simulink model "SIMbuckconverterPVmodel"  (R2020b)
settings: Solver=VariableStepAuto  StartTime=0.0  StopTime=3  RelTol=1e-3
libraries: powerlib x10, pid_lib x1, simulink x1
settings Model: SILPILModeSetting=veronly  ExtModeTrigDuration=2  Creator=colpari  LastModifiedBy=colpari
settings OptimizationCC: EnhancedBackFolding=on  PassReuseOutputArgsAs=Individual arguments  ZeroExternalMemoryAtStartup=off  ZeroInternalMemoryAtStartup=off  MaxStackSize=64  OptimizeBlockOrder=speed  DifferentSizesBufferReuse=on  OptimizationCustomize=off  EfficientTunableParamExpr=on
settings DebuggingCC: ParameterTunabilityLossMsg=error
settings HardwareCC: ProdBitPerInt=16  ProdBitPerPointer=16  ProdBitPerSizeT=16  ProdBitPerPtrDiffT=16  ProdLargestAtomicFloat=None  ProdWordSize=8  ProdHWDeviceType=Atmel->AVR  UseEmbeddedCoderFeatures=off
settings SFSimCC: MATLABDynamicMemAlloc=off
settings RTWCC: Description=Embedded Coder  SystemTargetFile=ert.tlc  HardwareBoard=Arduino Uno  TemplateMakefile=ert_default_tmf  Toolchain=Arduino AVR
settings CodeAppCC: ForceParamTrailComments=on  IgnoreCustomStorageClasses=off  OperatorAnnotations=on  SimulinkDataObjDesc=on  SFDataObjDesc=on  InsertBlockDesc=on
settings ERTTargetCC: SupportContinuousTime=on  SupportNonInlinedSFcns=on  SupportVariableSizeSignals=on  ExtModeStaticAllocSize=250
settings SimscapeCC: EditingMode=Restricted

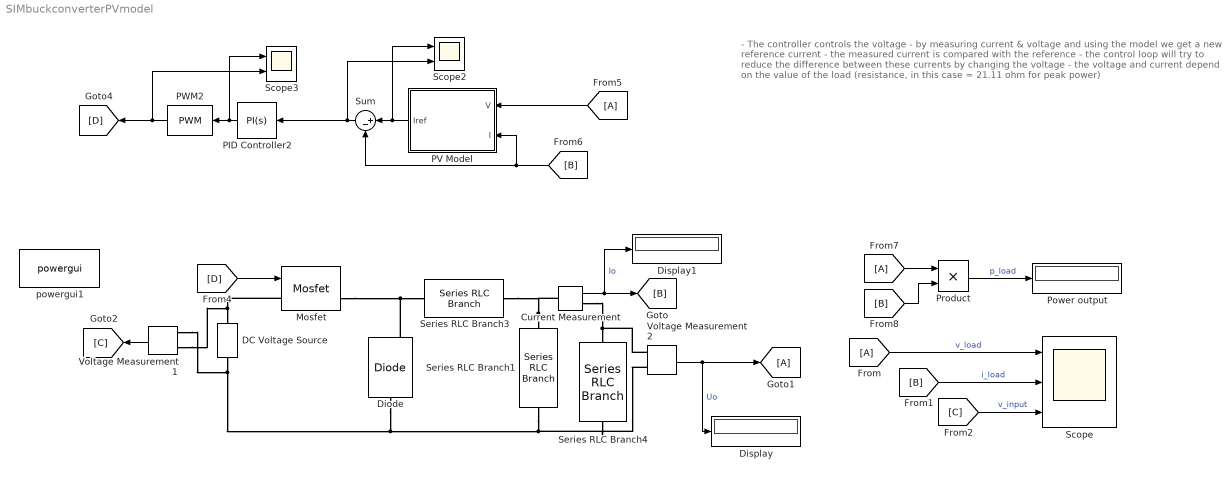
== system SIMbuckconverterPVmodel ==
  note: - The controller controls the voltage
      | - by measuring current & voltage and using the model we get a new reference current
      | - the measured current is compared with the reference
      | - the control loop will try to reduce the difference between these currents by changing the voltage
      | - the voltage and current depend on the value of the load (resistance, in this case = 21.11 ohm for peak power)
  Current Measurement : powerlib/Measurements/Current Measurement  PhasorSimulation=off  OutputType=Complex  PSBequivalent=0
  DC Voltage Source : powerlib/Electrical Sources/DC Voltage Source  Amplitude=12  Measurements=None
  Diode : powerlib/Power Electronics/Diode  Ron=0.001  Lon=0  Vf=0.8  IC=0  UseSnubber=0  Rs=500  Cs=250e-9  Measurements=on
  Display : Display
  Display1 : Display
  Mosfet : powerlib/Power Electronics/Mosfet  Ron=0.1  Lon=0  Rd=0.01  Vfd=0  IC=0  Rs=1e5  Cs=inf  Measurements=on
  PID Controller2 : pid_lib/PID Controller  Controller=PI  Form=Parallel  TimeDomain=Continuous-time  UseExternalTs=off  SampleTime=-1  IntegratorMethod=Forward Euler  FilterMethod=Forward Euler  ControllerParametersSource=internal  P=0.8  I=90  D=0  UseFilter=on  N=100  TunerSelectOption=Frequency Response Based  InitialConditionSource=internal  InitialConditionForIntegrator=0  InitialConditionForFilter=0  DifferentiatorICPrevScaledInput=0  ExternalReset=none  TrackingMode=off  Kt=1  LimitOutput=on  SatLimitsSource=internal  UpperSaturationLimit=0.99  LowerSaturationLimit=0.01  LinearizeAsGain=on  AntiWindupMode=none  Kb=1  RndMeth=Zero  POutMin=[]  POutMax=[]  IOutMin=[]  IOutMax=[]  DOutMin=[]  DOutMax=[]  NOutMin=[]  NOutMax=[]  SumOutMin=[]  SumOutMax=[]  SaturationOutMin=[]  SaturationOutMax=[]  PParamMin=[]  PParamMax=[]  IParamMin=[]  IParamMax=[]  DParamMin=[]  DParamMax=[]  NParamMin=[]  NParamMax=[]  KbParamMin=[]  KbParamMax=[]  KtParamMin=[]  KtParamMax=[]  KbOutMin=[]  KbOutMax=[]  KtOutMin=[]  KtOutMax=[]  IntegratorOutMin=[]  IntegratorOutMax=[]  FilterOutMin=[]  FilterOutMax=[]  SumI1OutMin=[]  SumI1OutMax=[]  SumI2OutMin=[]  SumI2OutMax=[]  SumI3OutMin=[]  SumI3OutMax=[]  SumI4OutMin=[]  SumI4OutMax=[]  SumDOutMin=[]  SumDOutMax=[]  DifferentiatorOutMin=[]  DifferentiatorOutMax=[]  FilterDiffOutCoefMin=[]  FilterDiffOutCoefMax=[]  ReciprocalOutMin=[]  ReciprocalOutMax=[]  SumDenOutMin=[]  SumDenOutMax=[]  SumNumOutMin=[]  SumNumOutMax=[]  DivideOutMin=[]  DivideOutMax=[]  UdiffTsProdOutMin=[]  UdiffTsProdOutMax=[]  NTsProdOutMin=[]  NTsProdOutMax=[]  UintegralTsProdOutMin=[]  UintegralTsProdOutMax=[]  UngainTsProdOutMin=[]  UngainTsProdOutMax=[]  IntegratorContinuousStateAttributes=''  IntegratorStateMustResolveToSignalObject=off  IntegratorRTWStateStorageClass=Auto  FilterContinuousStateAttributes=''  FilterStateMustResolveToSignalObject=off  FilterRTWStateStorageClass=Auto  ParallelPVariant=InternalParameters  IdealPVariant=Disabled  IVariant=InternalParameters  DVariant=Disabled  IntegratorVariant=Continuous  SatVariant=Enabled  AWVariant=Passthrough  PCopyVariant=Disabled  TRVariant=Disabled  FdbkBlocksVariant=Forward  IdealPFdbkVariant=Disabled  SatFdbkVariant=Disabled  DerivativeFilterVariant=Disabled  NVariant=Disabled  NCopyVariant=Disabled_SignalSpec  FilterICVariant=Disabled  IntegratorICVariant=InternalICs  ExternalResetVariant=Disabled  TRSumVariant=Passthrough  SumFdbkVariant=Disabled  SumVariant=Sum_PI  TsampFilterVariant=InternalTs  TsampNgainVariant=Passthrough  TsampIntegralVariant=Passthrough  ExternalSaturationOutDataTypeStr=Inherit: Same as second input
  PV Model : Subsystem
  PWM2 : simulink/Discontinuities/PWM  DisableCoverage=on  Period=1/3921.16  DisallowZeroDutyCycle=off  RunAtFixedTimeIntervals=on  SampleTime=0.00001
  Power output : Display
  Product : Product
  Scope : Scope  NumInputPorts=3
  Scope2 : Scope  NumInputPorts=2
  Scope3 : Scope  NumInputPorts=2
  Series RLC Branch1 : powerlib/Elements/Series RLC Branch  LConnTagsString=__new0  RConnTagsString=__new0  BranchType=C  Resistance=1  Inductance=1e-3  SetiL0=off  InitialCurrent=0  Capacitance=4700e-6  Setx0=off  InitialVoltage=0  Measurements=None
  Series RLC Branch3 : powerlib/Elements/Series RLC Branch  LConnTagsString=__new0  RConnTagsString=__new0  BranchType=L  Resistance=1  Inductance=1e-3  SetiL0=off  InitialCurrent=0  Capacitance=1e-6  Setx0=off  InitialVoltage=0  Measurements=None
  Series RLC Branch4 : powerlib/Elements/Series RLC Branch  LConnTagsString=__new0  RConnTagsString=__new0  BranchType=R  Resistance=21.11  Inductance=1e-3  SetiL0=off  InitialCurrent=0  Capacitance=1e-6  Setx0=off  InitialVoltage=0  Measurements=None
  Sum : Sum  Inputs=|+-
  Voltage Measurement1 : powerlib/Measurements/Voltage Measurement  PhasorSimulation=off  OutputType=Complex  PSBequivalent=0
  Voltage Measurement2 : powerlib/Measurements/Voltage Measurement  PhasorSimulation=off  OutputType=Complex  PSBequivalent=0
  powergui1 : powerlib/powergui  Priority=1  SimulationMode=Continuous  SampleTime=50e-6  frequency=60  Iterations=50  frequencyindice=0  Pbase=100e6  ErrMax=1e-4  UnitsV=kV  UnitsW=MW  buscounter=0  FunctionMessages=off  echomessages=off  EnableUseOfTLC=off  CurrentSourceSwitches=off  DisableSnubberDevices=off  DisableRonSwitches=off  DisableVfSwitches=off  DisplayEquations=off  AutomaticDiscreteSolvers=off  SolverType=Tustin/Backward Euler (TBE)  Interpol=off  ExternalGateDelay=off  methode=off  Ts=100  x0status=blocks  SPID=on  SwTol=0  HookPort=off  NonlinearTolerance=1e-4  nMaxIteration=100  ContinueOnMaxIteration=off  RestoreLinks=warning  ResistiveCurrentMeasurement=off  Frange=[0:2:500]  Ylog=off  Xlog=on  ShowGrid=off  save=off  variable=ZData  structure=0  ZoomFFT=off  StartTime=0.0  cycles=1  DisplayStyle=1  fundamental=60  FreqAxis=off  MaxFrequency=1000  frequencyindicesteady=1  RmsSteady=1  display=off
  wires:
  PV Model/1(Iref) -> Scope2/1, Sum/1
  Sum/1 -> PID Controller2/1, Scope2/2
  [B] -> Scope/2  "i_load"
  [D] -> Mosfet/1
  Current Measurement/1 -> Display1/1, [B]  "Io"
  Voltage Measurement2/1 -> Display/1, [A]  "Uo"
  Voltage Measurement1/1 -> [C]
  [C] -> Scope/3  "v_input"
  [A] -> Scope/1  "v_load"
  [A] -> PV Model/1(V)
  [B] -> Sum/2, PV Model/2(I)
  PID Controller2/1 -> Scope3/1, PWM2/1
  PWM2/1 -> Scope3/2, [D]
  [A] -> Product/1
  [B] -> Product/2
  Product/1 -> Power output/1  "p_load"
  connections:
  DC Voltage Source/LConn1 -- Series RLC Branch4/RConn1 -- Voltage Measurement2/LConn2 -- Series RLC Branch1/RConn1 -- Diode/LConn1 -- Voltage Measurement1/LConn2
  Diode/RConn1 -- Mosfet/RConn1 -- Series RLC Branch3/LConn1
  Series RLC Branch1/LConn1 -- Series RLC Branch3/RConn1 -- Current Measurement/LConn1
  Series RLC Branch4/LConn1 -- Current Measurement/RConn1 -- Voltage Measurement2/LConn1
  DC Voltage Source/RConn1 -- Mosfet/LConn1 -- Voltage Measurement1/LConn1

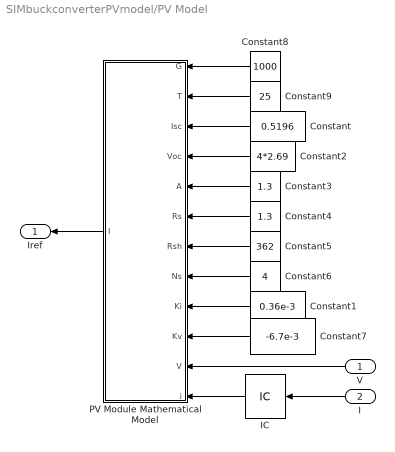
== system SIMbuckconverterPVmodel/PV Model ==
  V : Inport
  I : Inport  Port=2
  Constant : Constant  Value=0.5196
  Constant1 : Constant  Value=0.36e-3
  Constant2 : Constant  Value=4*2.69
  Constant3 : Constant  Value=1.3
  Constant4 : Constant  Value=1.3
  Constant5 : Constant  Value=362
  Constant6 : Constant  Value=4
  Constant7 : Constant  Value=-6.7e-3
  Constant8 : Constant  Value=1000
  Constant9 : Constant  Value=25
  IC : InitialCondition  Value=0
  PV Module Mathematical Model : MATLAB Function  TreatAsAtomicUnit=on
  Iref : Outport
  wires:
  Constant/1 -> PV Module Mathematical Model/3(Isc)
  Constant7/1 -> PV Module Mathematical Model/10(Kv)
  Constant5/1 -> PV Module Mathematical Model/7(Rsh)
  Constant6/1 -> PV Module Mathematical Model/8(Ns)
  Constant1/1 -> PV Module Mathematical Model/9(Ki)
  Constant8/1 -> PV Module Mathematical Model/1(G)
  Constant4/1 -> PV Module Mathematical Model/6(Rs)
  Constant2/1 -> PV Module Mathematical Model/4(Voc)
  Constant9/1 -> PV Module Mathematical Model/2(T)
  Constant3/1 -> PV Module Mathematical Model/5(A)
  PV Module Mathematical Model/1(I) -> Iref/1
  I/1 -> IC/1
  IC/1 -> PV Module Mathematical Model/12(i)
  V/1 -> PV Module Mathematical Model/11(V)

== matlab function SIMbuckconverterPVmodel/PV Model/PV Module Mathematical Model ==
  data: G input; T input; Isc input; Voc input; A input; Rs input; Rsh input; Ns input; Ki input; Kv input; V input; i input; I output
function I = fcn(G,T,Isc,Voc,A,Rs,Rsh,Ns,Ki,Kv,V,i)
    
    q = 1.6e-19;                          % Electron charge
    k = 1.38e-23;                         % Boltzmann constant
    Tcell = 273+T;                        % Cell temperature in Kelvin
    vt=(A*k*Tcell*Ns)/q;                  % Thermal voltage Equation(5)
        
    Isc_T = Isc+((Isc*(Ki/100))*(T-25));  % Isc temperature coef Equation(6)
    Voc_T = Voc+((Voc*(Kv/100))*(T-25));  % Voc temperature coef Equation(7)
    Is = Isc_T/(exp(Voc_T/vt)-1);         % Reverse saturation current Equation(8)
    Iph = Isc_T*(G/1000);                 % Photon current Equation(9)
    
    % Single diode model output current Equation(4)
    I = Iph-(Is*(exp((V+(i*Rs))/vt)-1))-((V+(i*Rs))/Rsh);
end
